simulink model "persist_test"  (R2025b)
settings: Solver=VariableStepAuto  StartTime=0.0  StopTime=10.0  RelTol=1e-3
settings Model: Creator=alokahn  LastModifiedBy=alokahn

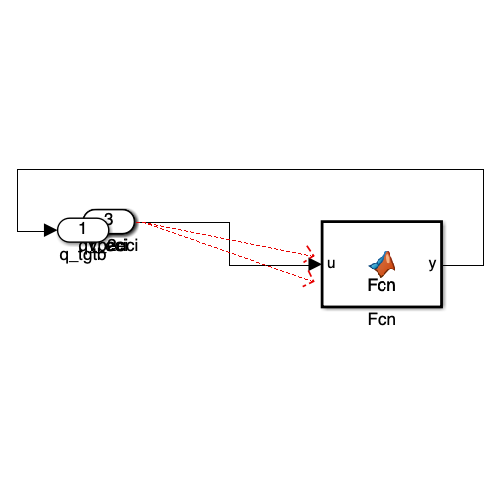
[thumbnail: Simulink's stored preview of the top-level diagram]
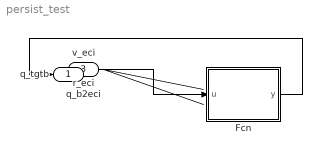
== system persist_test ==
  r_eci : Inport  PortDimensions=3
  v_eci : Inport  Port=2  PortDimensions=3
  q_b2eci : Inport  Port=3  PortDimensions=4
  Fcn : MATLAB Function  TreatAsAtomicUnit=on
  q_tgtb : Outport
  wires:
  r_eci/1 -> Fcn/1(u)
  v_eci/1 -> ?
  q_b2eci/1 -> ?
  Fcn/1(y) -> q_tgtb/1

== matlab function persist_test/Fcn ==
  data: u input; y output
function y = Fcn(u)
    if isempty(q_want_prev)
        q_want_prev = [1 0 0 0];
    end
    y = q_want_prev(1) + u;
end
